simulink model "BioReactor_model"  (R2022b)
settings: Solver=VariableStepAuto  StartTime=T_start  StopTime=T_stop  MaxStep=1e-1  RelTol=1e-3
undefined symbols (not defined in the file): K1, K2, muMAX, S_F, T_u, Tp, u_A, u_M, V, x1_0, x2_0, Y
libraries: simulink_extras x1
settings Model: Creator=gianfrancofenu  LastModifiedBy=gianfrancofenu
settings SolverCC: ShapePreserveControl=EnableAll
settings DataIOCC: SaveFormat=Array  SaveState=on  SignalLogging=off  DSMLogging=off

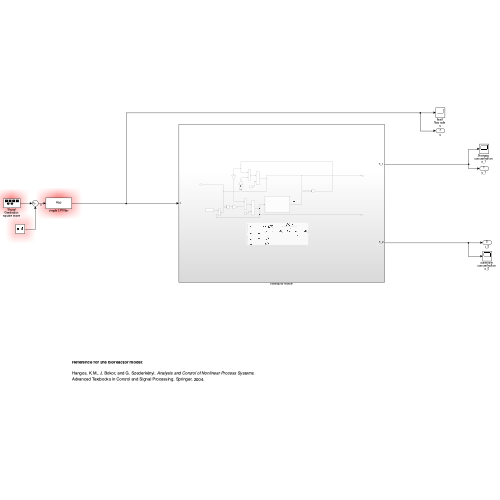
[thumbnail: Simulink's stored preview of the top-level diagram]
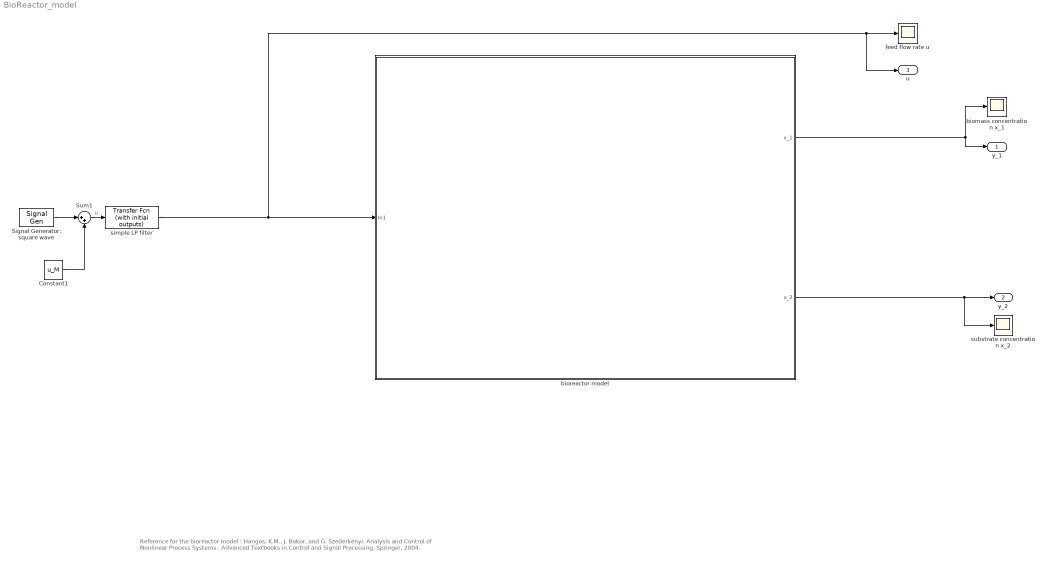
== system BioReactor_model ==
  note: Reference for the bioreactor model :
      |
      | Hangos, K.M., J. Bokor, and G. Szederkényi. Analysis and Control of Nonlinear Process Systems . Advanced Textbooks in Control and Signal Processing. Springer, 2004.
  Constant1 : Constant  Value=u_M  SampleTime=0
  Signal Generator: square wave : SignalGenerator  WaveForm=square  Amplitude=u_A  Frequency=1/T_u
  Sum1 : Sum  Inputs=|++
  biomass concentration x_1 : Scope
  bioreactor model : Subsystem
  feed flow rate u : Scope
  simple LP filter : simulink_extras/Additional Linear/Transfer Fcn (with initial outputs)  N=[1/Tp]  D="[1  1/Tp]"  Y0=u_M  U0=u_M
  substrate concentration x_2 : Scope
  y_1 : Outport
  y_2 : Outport  Port=2
  u : Outport  Port=3
  wires:
  Sum1/1 -> simple LP filter/1  "u"
  Signal Generator: square wave/1 -> Sum1/1
  Constant1/1 -> Sum1/2
  simple LP filter/1 -> u/1, feed flow rate u/1, bioreactor model/1(In1)
  bioreactor model/2(x_2) -> substrate concentration x_2/1, y_2/1
  bioreactor model/1(x_1) -> biomass concentration x_1/1, y_1/1

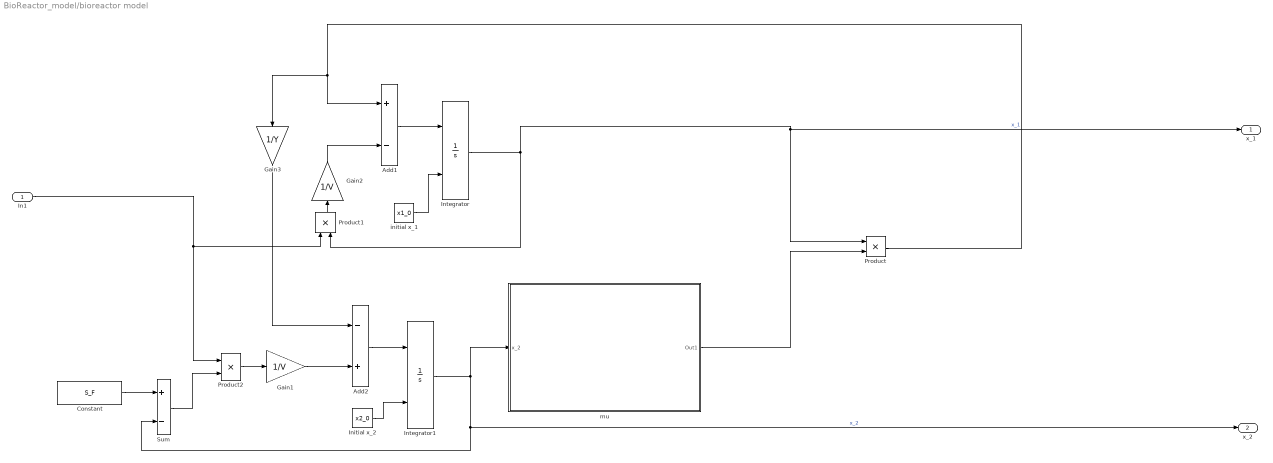
== system BioReactor_model/bioreactor model ==
  In1 : Inport
  Add1 : Sum  Inputs=+-
  Add2 : Sum  Inputs=-+
  Constant : Constant  Value=S_F  SampleTime=0
  Gain1 : Gain  Gain=1/V
  Gain2 : Gain  Gain=1/V
  Gain3 : Gain  Gain=1/Y
  Initial x_2 : Constant  Value=x2_0  SampleTime=0
  Integrator : Integrator  InitialConditionSource=external
  Integrator1 : Integrator  InitialConditionSource=external
  Product : Product
  Product1 : Product
  Product2 : Product
  Sum : Sum  Inputs=+-
  initial x_1 : Constant  Value=x1_0  SampleTime=0
  mu : Subsystem
  x_1 : Outport
  x_2 : Outport  Port=2
  wires:
  Add1/1 -> Integrator/1
  Integrator/1 -> x_1/1, Product/1, Product1/2  "x_1"
  Product2/1 -> Gain1/1
  initial x_1/1 -> Integrator/2
  mu/1(Out1) -> Product/2
  Gain3/1 -> Add2/1
  Product1/1 -> Gain2/1
  Initial x_2/1 -> Integrator1/2
  Constant/1 -> Sum/1
  Gain1/1 -> Add2/2
  Sum/1 -> Product2/2
  In1/1 -> Product2/1, Product1/1
  Product/1 -> Gain3/1, Add1/1
  Integrator1/1 -> mu/1(x_2), Sum/2, x_2/1  "x_2"
  Add2/1 -> Integrator1/1
  Gain2/1 -> Add1/2

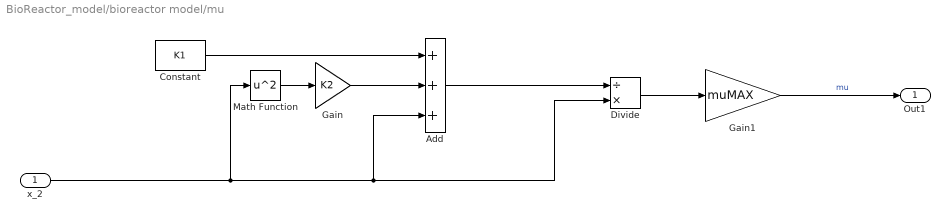
== system BioReactor_model/bioreactor model/mu ==
  x_2 : Inport
  Add : Sum  Inputs=+++
  Constant : Constant  Value=K1  SampleTime=0
  Divide : Product  Inputs=/*
  Gain : Gain  Gain=K2
  Gain1 : Gain  Gain=muMAX
  Math Function : Math  Operator=square
  Out1 : Outport
  wires:
  Constant/1 -> Add/1
  Gain/1 -> Add/2
  Add/1 -> Divide/1
  x_2/1 -> Math Function/1, Divide/2, Add/3
  Gain1/1 -> Out1/1  "mu"
  Divide/1 -> Gain1/1
  Math Function/1 -> Gain/1
